simulink model "Ej5_v5"  (R2015a)
settings: Solver=ode45  StartTime=0.0  StopTime=2  RelTol=1e-3
libraries: cstblocks x6, simulink x3
settings Model: Creator=Daniel  LastModifiedBy=Daniel

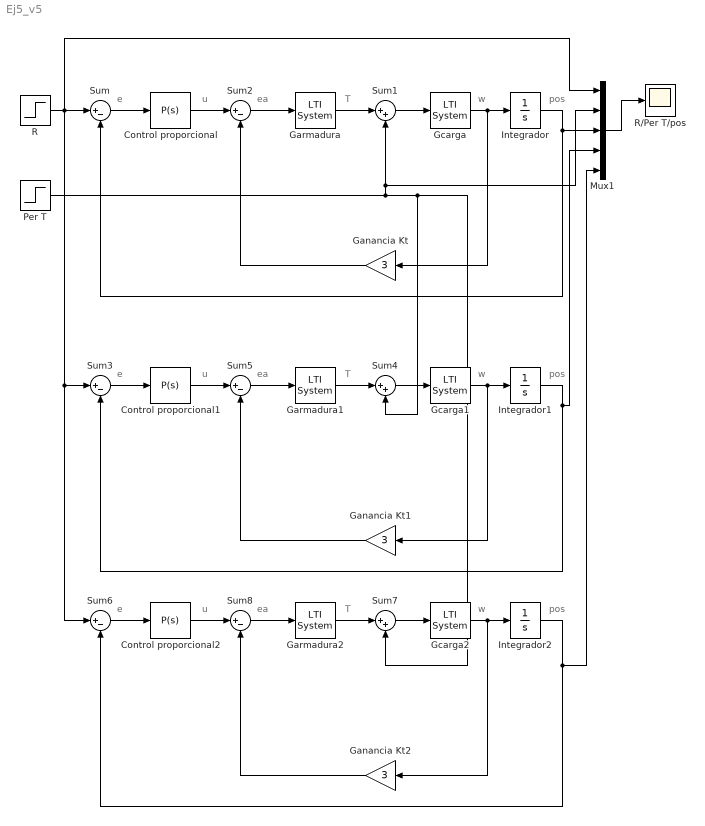
== system Ej5_v5 ==
  note: u
  note: T
  note: pos
  note: w
  note: e
  note: ea
  note: u
  note: T
  note: pos
  note: w
  note: e
  note: ea
  note: u
  note: T
  note: pos
  note: w
  note: e
  note: ea
  Control proporcional : simulink/Continuous/PID Controller  Controller=P  TimeDomain=Continuous-time  SampleTime=-1  IntegratorMethod=Forward Euler  FilterMethod=Forward Euler  Form=Ideal  UseFilter=on  ControllerParametersSource=internal  P=80  I=0  D=0.05  N=2000  InitialConditionSource=internal  InitialConditionForIntegrator=0  InitialConditionForFilter=0  ExternalReset=none  LimitOutput=off  UpperSaturationLimit=12  LowerSaturationLimit=-inf  LinearizeAsGain=on  AntiWindupMode=none  Kb=1  TrackingMode=off  Kt=1  PParamMin=[]  PParamMax=[]  IParamMin=[]  IParamMax=[]  DParamMin=[]  DParamMax=[]  NParamMin=[]  NParamMax=[]  KbParamMin=[]  KbParamMax=[]  KtParamMin=[]  KtParamMax=[]  POutMin=[]  POutMax=[]  IOutMin=[]  IOutMax=[]  DOutMin=[]  DOutMax=[]  NOutMin=[]  NOutMax=[]  KbOutMin=[]  KbOutMax=[]  KtOutMin=[]  KtOutMax=[]  IntegratorOutMin=[]  IntegratorOutMax=[]  FilterOutMin=[]  FilterOutMax=[]  SumOutMin=[]  SumOutMax=[]  SumI1OutMin=[]  SumI1OutMax=[]  SumI2OutMin=[]  SumI2OutMax=[]  SumI3OutMin=[]  SumI3OutMax=[]  SumDOutMin=[]  SumDOutMax=[]  SaturationOutMin=[]  SaturationOutMax=[]  IntegratorContinuousStateAttributes=''  IntegratorStateMustResolveToSignalObject=off  IntegratorRTWStateStorageClass=Auto  FilterContinuousStateAttributes=''  FilterStateMustResolveToSignalObject=off  FilterRTWStateStorageClass=Auto  DifferentiatorICPrevScaledInput=0  DifferentiatorOutMin=[]  DifferentiatorOutMax=[]
  Control proporcional1 : simulink/Continuous/PID Controller  Controller=P  TimeDomain=Continuous-time  SampleTime=-1  IntegratorMethod=Forward Euler  FilterMethod=Forward Euler  Form=Ideal  UseFilter=on  ControllerParametersSource=internal  P=100  I=0  D=0.05  N=2000  InitialConditionSource=internal  InitialConditionForIntegrator=0  InitialConditionForFilter=0  ExternalReset=none  LimitOutput=off  UpperSaturationLimit=12  LowerSaturationLimit=-inf  LinearizeAsGain=on  AntiWindupMode=none  Kb=1  TrackingMode=off  Kt=1  PParamMin=[]  PParamMax=[]  IParamMin=[]  IParamMax=[]  DParamMin=[]  DParamMax=[]  NParamMin=[]  NParamMax=[]  KbParamMin=[]  KbParamMax=[]  KtParamMin=[]  KtParamMax=[]  POutMin=[]  POutMax=[]  IOutMin=[]  IOutMax=[]  DOutMin=[]  DOutMax=[]  NOutMin=[]  NOutMax=[]  KbOutMin=[]  KbOutMax=[]  KtOutMin=[]  KtOutMax=[]  IntegratorOutMin=[]  IntegratorOutMax=[]  FilterOutMin=[]  FilterOutMax=[]  SumOutMin=[]  SumOutMax=[]  SumI1OutMin=[]  SumI1OutMax=[]  SumI2OutMin=[]  SumI2OutMax=[]  SumI3OutMin=[]  SumI3OutMax=[]  SumDOutMin=[]  SumDOutMax=[]  SaturationOutMin=[]  SaturationOutMax=[]  IntegratorContinuousStateAttributes=''  IntegratorStateMustResolveToSignalObject=off  IntegratorRTWStateStorageClass=Auto  FilterContinuousStateAttributes=''  FilterStateMustResolveToSignalObject=off  FilterRTWStateStorageClass=Auto  DifferentiatorICPrevScaledInput=0  DifferentiatorOutMin=[]  DifferentiatorOutMax=[]
  Control proporcional2 : simulink/Continuous/PID Controller  Controller=P  TimeDomain=Continuous-time  SampleTime=-1  IntegratorMethod=Forward Euler  FilterMethod=Forward Euler  Form=Ideal  UseFilter=on  ControllerParametersSource=internal  P=120  I=0  D=0.05  N=2000  InitialConditionSource=internal  InitialConditionForIntegrator=0  InitialConditionForFilter=0  ExternalReset=none  LimitOutput=off  UpperSaturationLimit=12  LowerSaturationLimit=-inf  LinearizeAsGain=on  AntiWindupMode=none  Kb=1  TrackingMode=off  Kt=1  PParamMin=[]  PParamMax=[]  IParamMin=[]  IParamMax=[]  DParamMin=[]  DParamMax=[]  NParamMin=[]  NParamMax=[]  KbParamMin=[]  KbParamMax=[]  KtParamMin=[]  KtParamMax=[]  POutMin=[]  POutMax=[]  IOutMin=[]  IOutMax=[]  DOutMin=[]  DOutMax=[]  NOutMin=[]  NOutMax=[]  KbOutMin=[]  KbOutMax=[]  KtOutMin=[]  KtOutMax=[]  IntegratorOutMin=[]  IntegratorOutMax=[]  FilterOutMin=[]  FilterOutMax=[]  SumOutMin=[]  SumOutMax=[]  SumI1OutMin=[]  SumI1OutMax=[]  SumI2OutMin=[]  SumI2OutMax=[]  SumI3OutMin=[]  SumI3OutMax=[]  SumDOutMin=[]  SumDOutMax=[]  SaturationOutMin=[]  SaturationOutMax=[]  IntegratorContinuousStateAttributes=''  IntegratorStateMustResolveToSignalObject=off  IntegratorRTWStateStorageClass=Auto  FilterContinuousStateAttributes=''  FilterStateMustResolveToSignalObject=off  FilterRTWStateStorageClass=Auto  DifferentiatorICPrevScaledInput=0  DifferentiatorOutMin=[]  DifferentiatorOutMax=[]
  Ganancia Kt : Gain  Gain=3
  Ganancia Kt1 : Gain  Gain=3
  Ganancia Kt2 : Gain  Gain=3
  Garmadura : cstblocks/LTI System  sys=Garm  IC=[]
  Garmadura1 : cstblocks/LTI System  sys=Garm  IC=[]
  Garmadura2 : cstblocks/LTI System  sys=Garm  IC=[]
  Gcarga : cstblocks/LTI System  sys=Gcar  IC=[]
  Gcarga1 : cstblocks/LTI System  sys=Gcar  IC=[]
  Gcarga2 : cstblocks/LTI System  sys=Gcar  IC=[]
  Integrador : Integrator
  Integrador1 : Integrator
  Integrador2 : Integrator
  Mux1 : Mux  Inputs=5
  Per T : Step  SampleTime=0
  R : Step  Time=0  After=0.6  SampleTime=0
  R/Per T/pos : Scope
      settings: SaveName=pos
  Sum{,2..3,5..6,8} (6 alike) : Sum  Inputs=|+-
  Sum1 : Sum  Inputs=|++
  Sum4 : Sum  Inputs=|++
  Sum7 : Sum  Inputs=|++
  wires:
  Sum/1 -> Control proporcional/1
  Mux1/1 -> R/Per T/pos/1
  Integrador/1 -> Mux1/3, Sum/2
  Garmadura/1 -> Sum1/1
  Sum1/1 -> Gcarga/1
  Control proporcional/1 -> Sum2/1
  Sum2/1 -> Garmadura/1
  Gcarga/1 -> Ganancia Kt/1, Integrador/1
  Ganancia Kt/1 -> Sum2/2
  Sum3/1 -> Control proporcional1/1
  Integrador1/1 -> Mux1/4, Sum3/2
  Garmadura1/1 -> Sum4/1
  Sum4/1 -> Gcarga1/1
  Control proporcional1/1 -> Sum5/1
  Sum5/1 -> Garmadura1/1
  Gcarga1/1 -> Ganancia Kt1/1, Integrador1/1
  Ganancia Kt1/1 -> Sum5/2
  Sum6/1 -> Control proporcional2/1
  Integrador2/1 -> Mux1/5, Sum6/2
  Garmadura2/1 -> Sum7/1
  Sum7/1 -> Gcarga2/1
  Per T/1 -> Sum7/2, Sum4/2, Sum1/2, Mux1/2
  Control proporcional2/1 -> Sum8/1
  Sum8/1 -> Garmadura2/1
  R/1 -> Sum6/1, Sum3/1, Mux1/1, Sum/1
  Gcarga2/1 -> Ganancia Kt2/1, Integrador2/1
  Ganancia Kt2/1 -> Sum8/2
